simulink model "Counter_Model"  (R2024a)
settings: Solver=VariableStepAuto  StartTime=0.0  StopTime=10.0  RelTol=1e-3
settings Model: Creator=DELL  LastModifiedBy=DELL

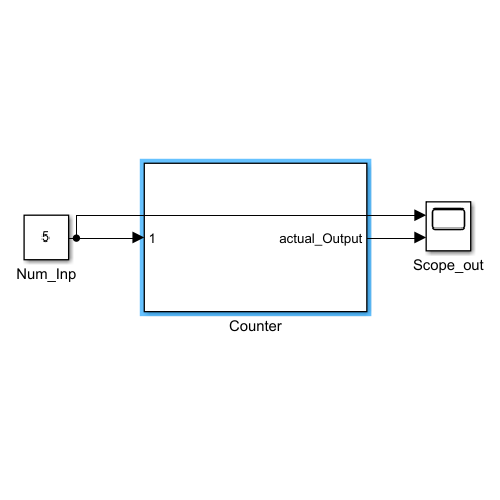
[thumbnail: Simulink's stored preview of the top-level diagram]
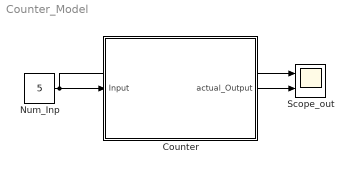
== system Counter_Model ==
  Counter : Subsystem
  Num_Inp : Constant  Value=5
  Scope_out : Scope  NumInputPorts=2
  wires:
  Num_Inp/1 -> Counter/1(Input), Scope_out/1
  Counter/1(actual_Output) -> Scope_out/2

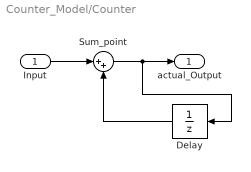
== system Counter_Model/Counter ==
  Input : Inport
  Delay : UnitDelay  SampleTime=-1  HasFrameUpgradeWarning=on
  Sum_point : Sum  Inputs=|++
  actual_Output : Outport
  wires:
  Input/1 -> Sum_point/1
  Sum_point/1 -> Delay/1, actual_Output/1
  Delay/1 -> Sum_point/2
